simulink model "Simulation_A"  (R2023b)
settings: Solver=VariableStepAuto  StartTime=0.0  StopTime=10.0  RelTol=1e-3
StopFcn:
  | show_res_simu('ref','speed')
undefined symbols (not defined in the file or in its folder): Bm, ke, kt, Ra, Su
libraries: Regulators_library x1, spspowerguiLib x1
settings Model: Creator=Student  LastModifiedBy=Student

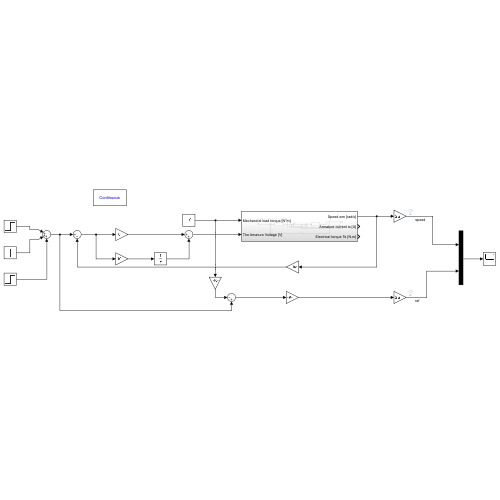
[thumbnail: Simulink's stored preview of the top-level diagram]
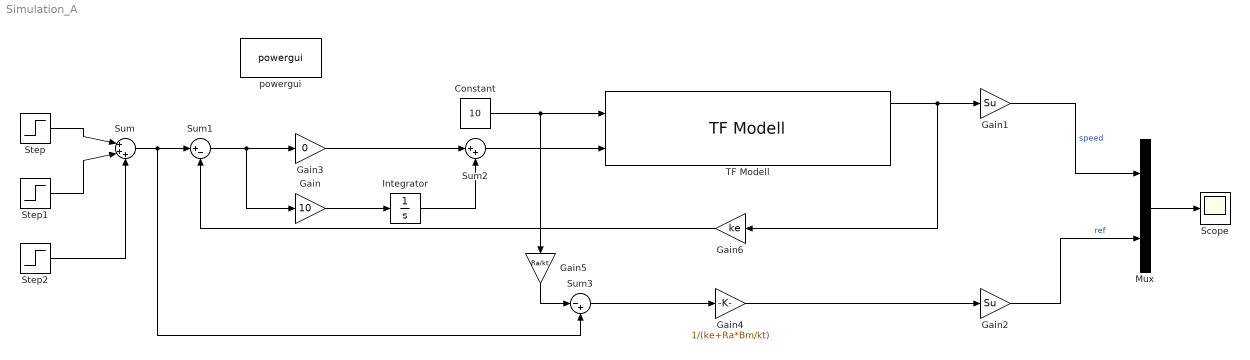
== system Simulation_A ==
  Constant : Constant  Value=10
  Gain : Gain  Gain=10
  Gain1 : Gain  Gain=Su
  Gain2 : Gain  Gain=Su
  Gain3 : Gain  Gain=0
  Gain4 : Gain  Gain=1/(ke+Ra*Bm/kt)
  Gain5 : Gain  Gain=Ra/kt
  Gain6 : Gain  Gain=ke
  Integrator : Integrator
  Mux : Mux  Inputs=2
  Scope : Scope
  Step : Step  Time=2.2  After=200  SampleTime=0
  Step1 : Step  Time=3.7  After=80  SampleTime=0
  Step2 : Step  Time=7.2  After=100  SampleTime=0
  Sum : Sum  Inputs=|+++
  Sum1 : Sum  Inputs=|+-
  Sum2 : Sum  Inputs=|++
  Sum3 : Sum  Inputs=|-+
  TF Modell : Regulators_library/TF Modell  SystemSampleTime=-1  VariantActivationTime=update diagram  AllowFlexibleInterface=on  Latency=0  AutoFrameSizeCalculation=off
  powergui : spspowerguiLib/powergui  Priority=1  SimulationMode=Continuous  SampleTime=50e-6  frequency=60  Iterations=50  frequencyindice=60  Pbase=100e6  ErrMax=1e-4  UnitsV=kV  UnitsW=MW  buscounter=0  FunctionMessages=off  echomessages=off  EnableUseOfTLC=off  CurrentSourceSwitches=off  DisableSnubberDevices=off  DisableRonSwitches=off  DisableVfSwitches=off  DisplayEquations=off  AutomaticDiscreteSolvers=off  SolverType=Tustin/Backward Euler (TBE)  Interpol=off  ExternalGateDelay=off  methode=off  Ts=100  x0status=blocks  SPID=on  SwTol=0  HookPort=off  NonlinearTolerance=1e-4  nMaxIteration=100  ContinueOnMaxIteration=off  RestoreLinks=warning  ResistiveCurrentMeasurement=off  Frange=[0:2:500]  Ylog=off  Xlog=on  ShowGrid=off  save=off  variable=ZData  structure=0  ZoomFFT=off  StartTime=0.0  cycles=1  DisplayStyle=1  fundamental=60  FreqAxis=off  MaxFrequency=1000  frequencyindicesteady=1  RmsSteady=1  display=off
  wires:
  Step/1 -> Sum/1
  Step1/1 -> Sum/2
  Step2/1 -> Sum/3
  Sum/1 -> Sum3/2, Sum1/1
  Sum1/1 -> Gain/1, Gain3/1
  Gain/1 -> Integrator/1
  Gain3/1 -> Sum2/1
  Integrator/1 -> Sum2/2
  Sum2/1 -> TF Modell/2
  Constant/1 -> TF Modell/1, Gain5/1
  TF Modell/1 -> Gain6/1, Gain1/1
  Gain1/1 -> Mux/1  "speed"
  Gain2/1 -> Mux/2  "ref"
  Gain5/1 -> Sum3/1
  Sum3/1 -> Gain4/1
  Gain4/1 -> Gain2/1
  Gain6/1 -> Sum1/2
  Mux/1 -> Scope/1
